simulink model "ex_41"  (R2018b)
settings: Solver=VariableStepAuto  StartTime=0.0  StopTime=5  RelTol=1e-3
settings Model: Creator=lenovo  LastModifiedBy=QJ-
settings DebuggingCC: LibraryContextMissingDiagnostic=none
settings SFSimCC: SimUseLocalCustomCode=off
settings RTWCC: RTWUseLocalCustomCode=off

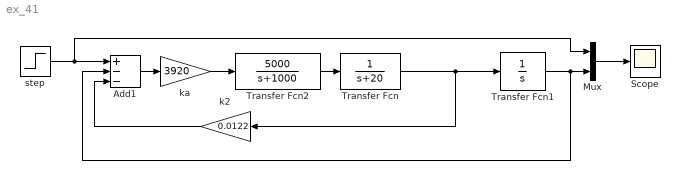
== system ex_41 ==
  Add1 : Sum  Inputs=+--
  Mux : Mux  Inputs=2
  Scope : Scope
  Transfer Fcn : TransferFcn  Denominator=[1 20]
  Transfer Fcn1 : TransferFcn  Denominator=[1 0]
  Transfer Fcn2 : TransferFcn  Numerator=[5000]  Denominator=[1 1000]
  k2 : Gain  Gain=0.0122
  ka : Gain  Gain=3920
  step : Step  SampleTime=1  mask(DiscretizedSource){}
      mask init:
      | %zoh
  wires:
  Mux/1 -> Scope/1
  Add1/1 -> ka/1
  k2/1 -> Add1/3
  ka/1 -> Transfer Fcn2/1
  Transfer Fcn/1 -> Transfer Fcn1/1, k2/1
  step/1 -> Mux/1, Add1/1
  Transfer Fcn1/1 -> Mux/2, Add1/2
  Transfer Fcn2/1 -> Transfer Fcn/1
